simulink model "testTriggerBuffer"  (R2014a)
settings: Solver=FixedStepDiscrete  StartTime=0.0  StopTime=Inf  FixedStep=0.001  RelTol=1e-3
undefined symbols (not defined in the file or in its folder): TaskEvent
libraries: simulink x1
settings Model: BufferReuse=off  Creator=djoshea  LastModifiedBy=djoshea
settings SolverCC: EnableConcurrentExecution=on
settings OptimizationCC: BlockReduction=off  OptimizeBlockIOStorage=off  BufferReuse=off  GlobalBufferReuse=off  ExpressionFolding=off  LocalBlockOutputs=off
settings HardwareCC: ProdIntDivRoundTo=Zero  ProdEndianess=LittleEndian  ProdHWDeviceType=Generic->32-bit x86 compatible
settings RTWCC: SystemTargetFile=slrt.tlc  TemplateMakefile=slrt_default_tmf  Description=Simulink Real-Time  ProcessScript=slrt_make_rtw_hook  RTWCompilerOptimization=On
settings SimulinkRealTimeCC: GeneratePreprocessorConditionals=Disable all  EnableShiftOperators=on

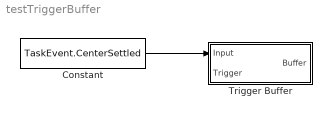
== system testTriggerBuffer ==
  Constant : Constant  Value=TaskEvent.CenterSettled
  Trigger Buffer : Subsystem  mask(Trigger Buffer){bufferSize=10, bufferType=Inherit: Same as input}
      mask prompts: bufferSize "Buffer Size (elements)"; bufferType "Content Type (specify enum if enum type)"
      mask help: This block concatenates all inputs it receives via a function-call trigger, with the output reflecting the concatenated inputs recevied during each single tick.
      mask init:
      | BusSerialize.maskUpdateTriggerBuffer(gcb);
  wires:
  Constant/1 -> Trigger Buffer/1(Input)

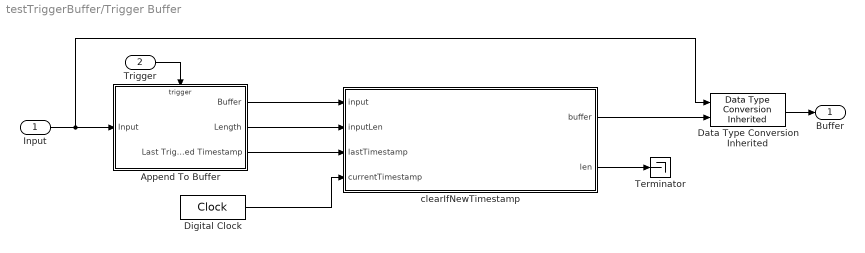
== system testTriggerBuffer/Trigger Buffer ==
  Input : Inport
  Trigger : Inport  Port=2
  Append To Buffer : Subsystem
  Data Type Conversion Inherited : simulink/Signal Attributes/Data Type Conversion Inherited  ConvertRealWorld=Real World Value  DoSatur=off
  Digital Clock : DigitalClock  SampleTime=-1
  Terminator : Terminator
  clearIfNewTimestamp : MATLAB Function  TreatAsAtomicUnit=on
  Buffer : Outport
  wires:
  clearIfNewTimestamp/2(len) -> Terminator/1
  Input/1 -> Data Type Conversion Inherited/1, Append To Buffer/1(Input)
  Append To Buffer/3(Last Triggered Timestamp) -> clearIfNewTimestamp/3(lastTimestamp)
  Append To Buffer/2(Length) -> clearIfNewTimestamp/2(inputLen)
  Append To Buffer/1(Buffer) -> clearIfNewTimestamp/1(input)
  Digital Clock/1 -> clearIfNewTimestamp/4(currentTimestamp)
  Trigger/1 -> Append To Buffer/Trigger
  Data Type Conversion Inherited/1 -> Buffer/1
  clearIfNewTimestamp/1(buffer) -> Data Type Conversion Inherited/2

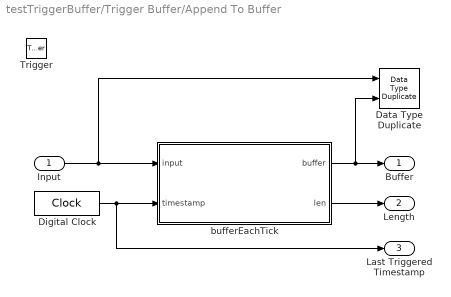
== system testTriggerBuffer/Trigger Buffer/Append To Buffer ==
  Input : Inport
  Trigger : TriggerPort  TriggerType=function-call  StatesWhenEnabling=reset  PortDimensions=1
  Data Type Duplicate : DataTypeDuplicate
  Digital Clock : DigitalClock  SampleTime=-1
  bufferEachTick : MATLAB Function  TreatAsAtomicUnit=on
  Buffer : Outport
  Length : Outport  Port=2
  Last Triggered Timestamp : Outport  Port=3
  wires:
  Digital Clock/1 -> bufferEachTick/2(timestamp), Last Triggered Timestamp/1
  Input/1 -> bufferEachTick/1(input), Data Type Duplicate/1
  bufferEachTick/1(buffer) -> Buffer/1, Data Type Duplicate/2
  bufferEachTick/2(len) -> Length/1

== matlab function testTriggerBuffer/Trigger Buffer/clearIfNewTimestamp ==
  data: input input size=bufferSize; inputLen input uint32 size=1; buffer output size=bufferSize; lastTimestamp input; currentTimestamp input size=1; len output uint32 size=1
function [buffer, len]   = clearIfNewTimestamp(input, inputLen, lastTimestamp, currentTimestamp)
%#codegen

if lastTimestamp == currentTimestamp
    buffer = input;
    len = inputLen;
else
    buffer = zeros(0, 1, class(input));
    len = zeros(1, 1, class(inputLen)); %#ok<ZEROLIKE>
end

== matlab function testTriggerBuffer/Trigger Buffer/Append To Buffer/bufferEachTick ==
  data: input input; buffer output size=bufferSize; timestamp input; len output uint32 size=1; bufferSize parameter size=1
function [buffer, len] = bufferEachTick(input, timestamp, bufferSize)
%#codegen

persistent pBuffer;
persistent pLastTimestamp;

coder.varsize('pBuffer', bufferSize, true);

clear = uint8(0);

% initialize persistents
if isempty(pBuffer) || isempty(pLastTimestamp)
    pBuffer = zeros(0, 1, class(input)); %#ok<ZEROLIKE>
    pLastTimestamp = timestamp;
end

% determine if this is a new tick and reset the output if it is
if pLastTimestamp ~= timestamp
    pLastTimestamp = timestamp;
    clear = uint8(1);
end

if clear
    pBuffer = input(:);
elseif numel(pBuffer) == 0
    pBuffer = input(:);
elseif numel(pBuffer) + numel(input) < bufferSize
    pBuffer = [pBuffer; input(:)];
end

buffer = pBuffer;
len = uint32(numel(buffer));
